simulink model "motorconfigmat"  (R2023b)
settings: Solver=VariableStepAuto  StartTime=0.0  StopTime=30  RelTol=1e-3
InitFcn:
  | Kpz = 0.3 ;
  | KIz = 0;
  | 
  | bh = 0.010290;  % batan hacim m^3
  | m = 10.5     ;  % aracın kütlesi kg
  | g = 9.81     ;  % yer çekimi ivmesi
  | p = 1000     ; % kg / m^3 yogunluk
  | W = m*g      ;  % aracın agırlıgı N
  | B = p*g*bh   ;  % Kaldırma kuvveti  N
  | 
  | xg = 0 ; % rgid body frame e göre ağırlık merkzi kordinatları
  | yg = 0 ;
  | zg = 0.02 ;
  | 
  | Ix = 0.1011 ; % kg *  m ^2
  | Iy = 0.1159 ;
  | Iz = 0.1615 ;
  | 
  | thrustCoefficient = 50/21.5 ;
  | 
  | % Add mass parametreleri
  | Xu_dot = -5.5;   % Surge direction
  | Yv_dot = -12.7;  % Sway direction
  | Zw_dot = -14.57; % Heave direction
  | 
  | Kp_dot = -0.12;  % Roll moment
  | Mq_dot = -0.12;  % Pitch moment
  | Nr_dot = -0.12;  % Yaw moment
  | 
  | % Linear Damping Values (Doğrusal Sönümleme Katsayıları)
  | Xu = -4.03;   % Ns/m
  | Yv = -6.22;   % Ns/m
  | Zw = -5.18;   % Ns/m
  | Kp = -0.07;   % Ns/rad
  | Mq = -0.07;   % Ns/rad
  | Nr = -0.07;   % Ns/rad
  | 
  | % Quadratic Damping Values (Doğrusal Olmayan Sönümleme Katsayıları)
  | Xuu = -18.18;  % Ns^2/m^2
  | Yvv = -21.66;  % Ns^2/m^2
  | Zww = -36.99;  % Ns^2/m^2
  | Kpp = -1.55;   % Ns^2/rad^2
  | Mqq = -1.55;   % Ns^2/rad^2
  | Nrr = -1.55;   % Ns^2/rad^2
undefined symbols (not defined in the file or in its folder): X, Y, Z
libraries: slpidlib x11, nesl_utility x7, sm_lib x6, fuzblock x1
(part 1 of 2)
settings Model: Creator=Yaser  LastModifiedBy=User

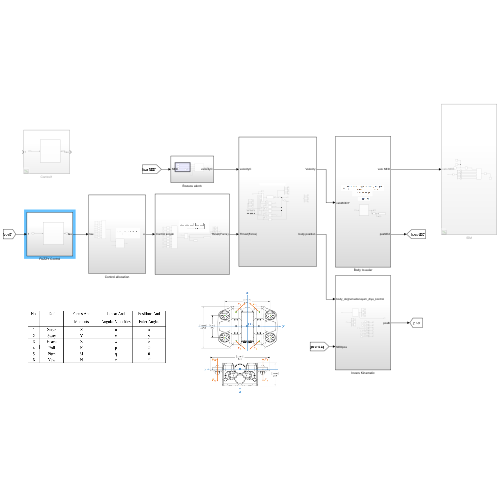
[thumbnail: Simulink's stored preview of the top-level diagram]
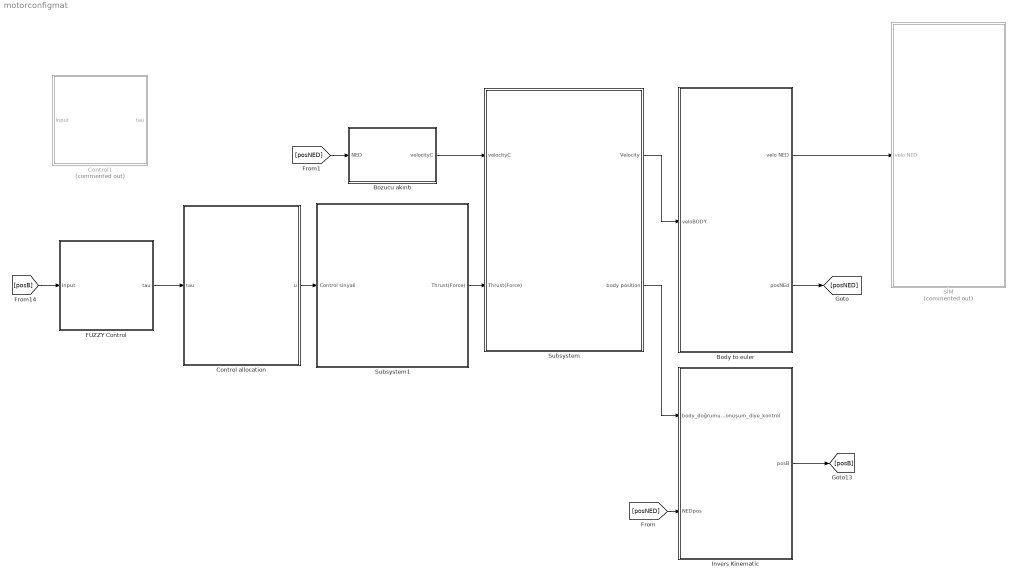
== system motorconfigmat ==
  Body to euler : Subsystem
  Bozucu akıntı : Subsystem
  Control allocation : Subsystem
  Control1 : Subsystem  Commented=on
  FUZZY Control : Subsystem
  Invers Kinematic : Subsystem
  Subsystem : Subsystem
  Subsystem1 : Subsystem
  SİM : Subsystem  Commented=on
  wires:
  [posNED] -> Invers Kinematic/2(NEDpos)
  Subsystem/2(body position) -> Invers Kinematic/1(body_doğrumudonuşum_diye_kontrol)
  Body to euler/2(posNEd) -> [posNED]
  [posB] -> FUZZY Control/1(Input)
  Subsystem/1(Velocity) -> Body to euler/1(veloBODY)
  Bozucu akıntı/1(velocityC) -> Subsystem/1(velocityC)
  Body to euler/1(velo NED) -> SİM/1(velo NED)
  Invers Kinematic/1(posB) -> [posB]
  Subsystem1/1(Thrust(Force)) -> Subsystem/2(Thrust(Force))
  FUZZY Control/1(tau) -> Control allocation/1(tau)
  Control allocation/1(u) -> Subsystem1/1(Control sinyali)
  [posNED] -> Bozucu akıntı/1(NED)

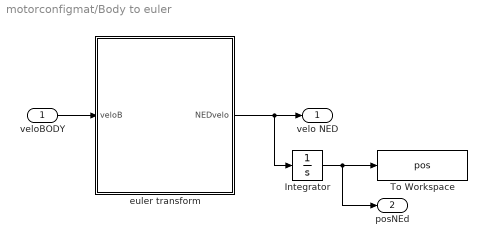
== system motorconfigmat/Body to euler ==
  veloBODY : Inport
  Integrator : Integrator
  To Workspace : ToWorkspace  VariableName=pos  SaveFormat=Timeseries  SampleTime=-1
  euler transform : MATLAB Function  TreatAsAtomicUnit=on
  velo NED : Outport
  posNEd : Outport  Port=2
  wires:
  veloBODY/1 -> euler transform/1(veloB)
  euler transform/1(NEDvelo) -> Integrator/1, velo NED/1
  Integrator/1 -> To Workspace/1, posNEd/1

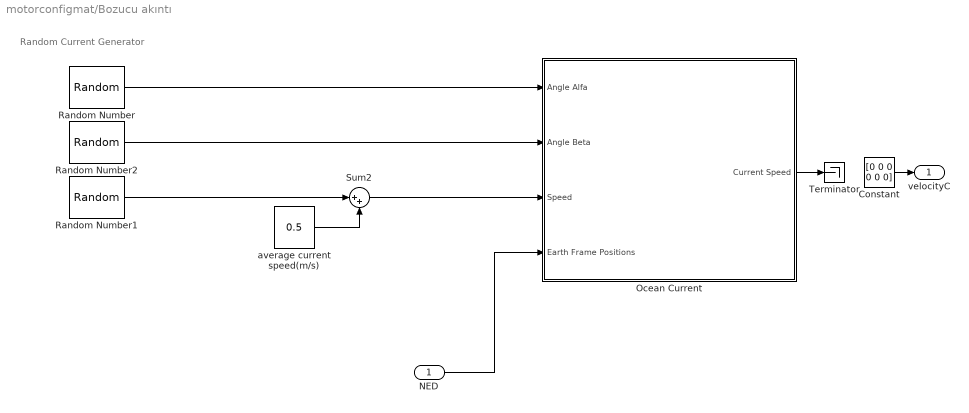
== system motorconfigmat/Bozucu akıntı ==
  note: Random Current Generator
  NED : Inport
  Constant : Constant  Value=[0 0 0 0 0 0]
  Ocean Current : Subsystem
  Random Number : RandomNumber  Mean=45  Variance=45  Seed=1  SampleTime=5
  Random Number1 : RandomNumber  Variance=0.02  Seed=0.025  SampleTime=5
  Random Number2 : RandomNumber  Mean=45  Variance=45  Seed=1  SampleTime=5
  Sum2 : Sum  Inputs=|++
  Terminator : Terminator
  average current speed(m/s) : Constant  Value=0.5
  velocityC : Outport
  wires:
  Random Number1/1 -> Sum2/1
  Random Number/1 -> Ocean Current/1(Angle Alfa)
  average current speed(m/s)/1 -> Sum2/2
  Sum2/1 -> Ocean Current/3(Speed)
  Random Number2/1 -> Ocean Current/2(Angle Beta)
  NED/1 -> Ocean Current/4(Earth Frame Positions)
  Ocean Current/1(Current Speed) -> Terminator/1
  Constant/1 -> velocityC/1

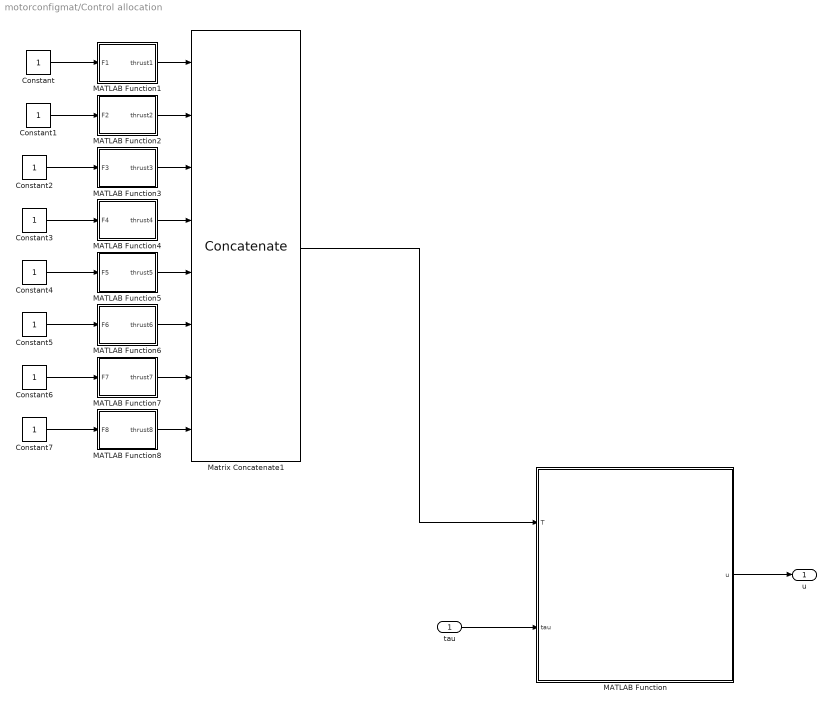
== system motorconfigmat/Control allocation ==
  tau : Inport
  Constant{,1..7} (8 alike) : Constant
  MATLAB Function : MATLAB Function  TreatAsAtomicUnit=on
  MATLAB Function1 : MATLAB Function  TreatAsAtomicUnit=on
  MATLAB Function2 : MATLAB Function  TreatAsAtomicUnit=on
  MATLAB Function3 : MATLAB Function  TreatAsAtomicUnit=on
  MATLAB Function4 : MATLAB Function  TreatAsAtomicUnit=on
  MATLAB Function5 : MATLAB Function  TreatAsAtomicUnit=on
  MATLAB Function6 : MATLAB Function  TreatAsAtomicUnit=on
  MATLAB Function7 : MATLAB Function  TreatAsAtomicUnit=on
  MATLAB Function8 : MATLAB Function  TreatAsAtomicUnit=on
  Matrix Concatenate1 : Concatenate  NumInputs=8  Mode=Multidimensional array  ConcatenateDimension=2
  u : Outport
  wires:
  MATLAB Function/1(u) -> u/1
  tau/1 -> MATLAB Function/2(tau)
  MATLAB Function4/1(thrust4) -> Matrix Concatenate1/4
  Constant/1 -> MATLAB Function1/1(F1)
  MATLAB Function2/1(thrust2) -> Matrix Concatenate1/2
  Constant6/1 -> MATLAB Function7/1(F7)
  MATLAB Function6/1(thrust6) -> Matrix Concatenate1/6
  MATLAB Function8/1(thrust8) -> Matrix Concatenate1/8
  Constant5/1 -> MATLAB Function6/1(F6)
  MATLAB Function7/1(thrust7) -> Matrix Concatenate1/7
  Constant4/1 -> MATLAB Function5/1(F5)
  Constant3/1 -> MATLAB Function4/1(F4)
  Constant7/1 -> MATLAB Function8/1(F8)
  MATLAB Function5/1(thrust5) -> Matrix Concatenate1/5
  Constant2/1 -> MATLAB Function3/1(F3)
  MATLAB Function3/1(thrust3) -> Matrix Concatenate1/3
  MATLAB Function1/1(thrust1) -> Matrix Concatenate1/1
  Constant1/1 -> MATLAB Function2/1(F2)
  Matrix Concatenate1/1 -> MATLAB Function/1(T)

== system motorconfigmat/Control1 ==
  Input : Inport
  divecont1 : Subsystem
  tau : Outport
  wires:
  divecont1/1(Out1) -> tau/1
  Input/1 -> divecont1/1(Input)

== system motorconfigmat/FUZZY Control ==
  Input : Inport
  divecont1 : Subsystem
  tau : Outport
  wires:
  Input/1 -> divecont1/1(Input)
  divecont1/1(Out1) -> tau/1

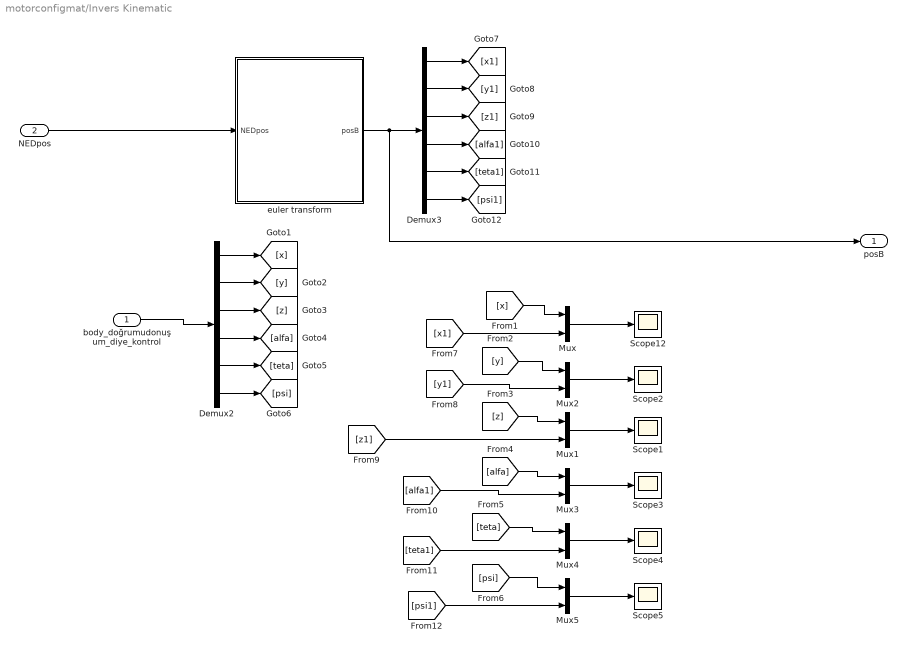
== system motorconfigmat/Invers Kinematic ==
  body_doğrumudonuşum_diye_kontrol : Inport
  NEDpos : Inport  Port=2
  Demux2 : Demux  Outputs=6
  Demux3 : Demux  Outputs=6
  Mux{,1..5} (6 alike) : Mux  Inputs=2
  Scope{1..5,12} (6 alike) : Scope
  euler transform : MATLAB Function  TreatAsAtomicUnit=on
  posB : Outport
  wires:
  [psi1] -> Mux5/2
  body_doğrumudonuşum_diye_kontrol/1 -> Demux2/1
  [x1] -> Mux/2
  Mux4/1 -> Scope4/1
  [z] -> Mux1/1
  euler transform/1(posB) -> posB/1, Demux3/1
  Demux3/1 -> [x1]
  Demux3/4 -> [alfa1]
  Demux3/5 -> [teta1]
  [z1] -> Mux1/2
  [y1] -> Mux2/2
  Mux3/1 -> Scope3/1
  [x] -> Mux/1
  Demux2/5 -> [teta]
  [psi] -> Mux5/1
  Demux3/6 -> [psi1]
  [alfa1] -> Mux3/2
  [teta1] -> Mux4/2
  [alfa] -> Mux3/1
  [teta] -> Mux4/1
  Mux2/1 -> Scope2/1
  Demux3/2 -> [y1]
  Demux2/1 -> [x]
  Mux1/1 -> Scope1/1
  [y] -> Mux2/1
  Demux3/3 -> [z1]
  Demux2/3 -> [z]
  Mux5/1 -> Scope5/1
  NEDpos/1 -> euler transform/1(NEDpos)
  Demux2/2 -> [y]
  Demux2/6 -> [psi]
  Mux/1 -> Scope12/1
  Demux2/4 -> [alfa]

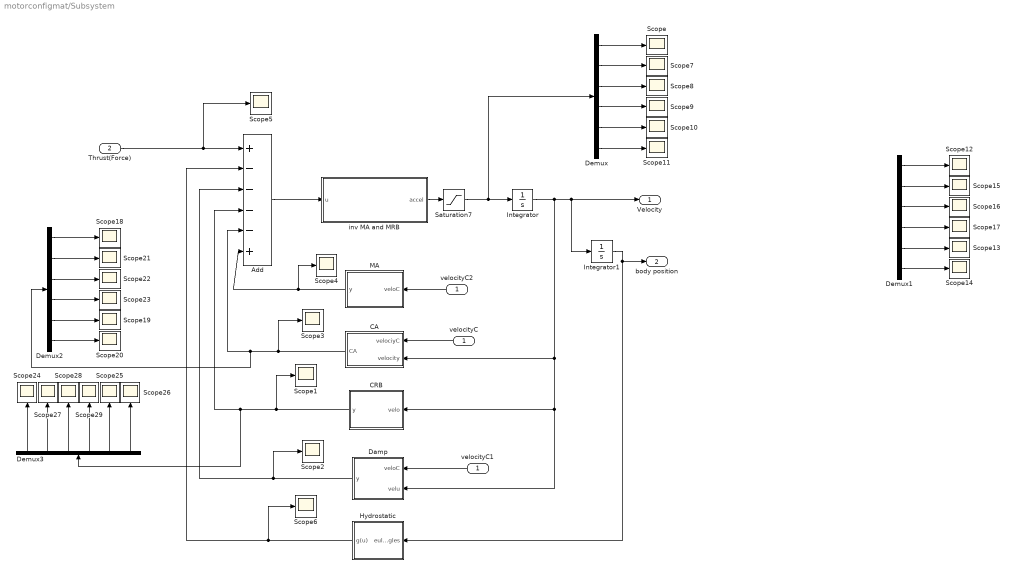
== system motorconfigmat/Subsystem ==
  velocityC : Inport
  Thrust(Force) : Inport  Port=2
  Add : Sum  Inputs=+----+
  CA : Subsystem
  CRB : Subsystem
  Damp : Subsystem
  Demux{,1..3} (4 alike) : Demux  Outputs=6
  Hydrostatic : Subsystem
  Integrator : Integrator
  Integrator1 : Integrator
  MA : Subsystem
  Saturation7 : Saturate  UpperLimit=1000  LowerLimit=-100
  Scope{,1..29} (30 alike) : Scope
  inv MA and MRB : Subsystem
  velocityC1 : InportShadow
  velocityC2 : InportShadow
  Velocity : Outport
  body position : Outport  Port=2
  wires:
  CA/1(CA) -> Scope3/1, Demux2/1, Add/5
  CRB/1(y) -> Scope1/1, Demux3/1, Add/4
  Integrator1/1 -> body position/1, Hydrostatic/1(euler angles)
  Add/1 -> inv MA and MRB/1(u)
  Integrator/1 -> Integrator1/1, Velocity/1, Damp/2(velu), CRB/1(velo), CA/2(velocity)
  Hydrostatic/1(g(u)) -> Scope6/1, Add/2
  Damp/1(y) -> Scope2/1, Add/3
  velocityC/1 -> CA/1(velociyC)
  velocityC1/1 -> Damp/1(veloC)
  velocityC2/1 -> MA/1(veloC)
  MA/1(y) -> Scope4/1, Add/6
  inv MA and MRB/1(accel) -> Saturation7/1
  Saturation7/1 -> Demux/1, Integrator/1
  Thrust(Force)/1 -> Scope5/1, Add/1
  Demux/1 -> Scope/1
  Demux/2 -> Scope7/1
  Demux/3 -> Scope8/1
  Demux/4 -> Scope9/1
  Demux/5 -> Scope10/1
  Demux/6 -> Scope11/1
  Demux1/1 -> Scope12/1
  Demux1/3 -> Scope16/1
  Demux1/6 -> Scope14/1
  Demux1/2 -> Scope15/1
  Demux1/4 -> Scope17/1
  Demux1/5 -> Scope13/1
  Demux2/1 -> Scope18/1
  Demux2/4 -> Scope23/1
  Demux2/2 -> Scope21/1
  Demux2/3 -> Scope22/1
  Demux2/5 -> Scope19/1
  Demux2/6 -> Scope20/1
  Demux3/5 -> Scope25/1
  Demux3/3 -> Scope28/1
  Demux3/2 -> Scope27/1
  Demux3/1 -> Scope24/1
  Demux3/4 -> Scope29/1
  Demux3/6 -> Scope26/1

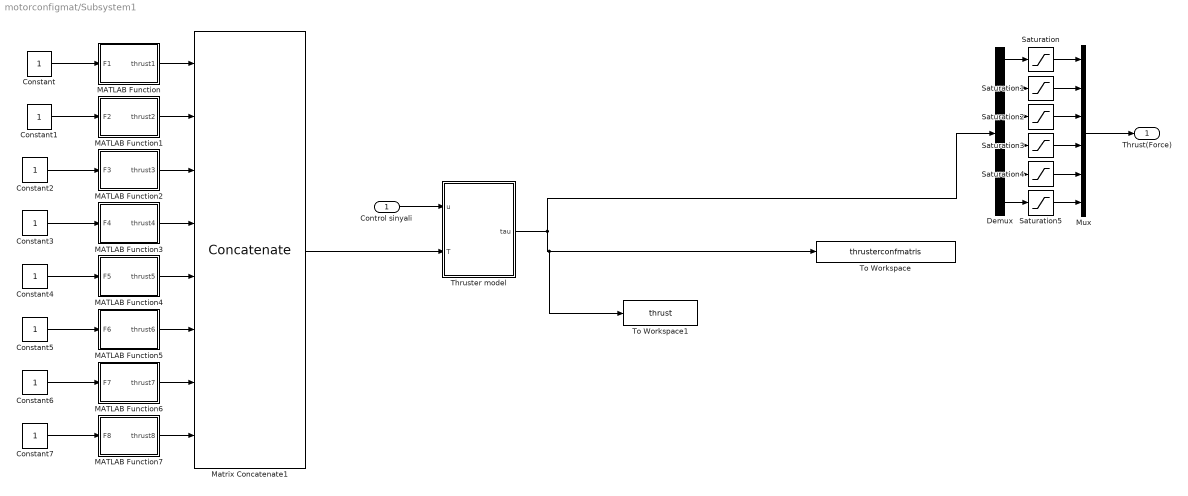
== system motorconfigmat/Subsystem1 ==
  Control sinyali : Inport
  Constant{,1..7} (8 alike) : Constant
  Demux : Demux  Outputs=6
  MATLAB Function : MATLAB Function  TreatAsAtomicUnit=on
  MATLAB Function1 : MATLAB Function  TreatAsAtomicUnit=on
  MATLAB Function2 : MATLAB Function  TreatAsAtomicUnit=on
  MATLAB Function3 : MATLAB Function  TreatAsAtomicUnit=on
  MATLAB Function4 : MATLAB Function  TreatAsAtomicUnit=on
  MATLAB Function5 : MATLAB Function  TreatAsAtomicUnit=on
  MATLAB Function6 : MATLAB Function  TreatAsAtomicUnit=on
  MATLAB Function7 : MATLAB Function  TreatAsAtomicUnit=on
  Matrix Concatenate1 : Concatenate  NumInputs=8  Mode=Multidimensional array  ConcatenateDimension=2
  Mux : Mux  Inputs=6
  Saturation : Saturate  UpperLimit=40*0.707*4  LowerLimit=-40*0.707*4
  Saturation1 : Saturate  UpperLimit=40*0.707*4  LowerLimit=-40*0.707*4
  Saturation2 : Saturate  UpperLimit=40*4  LowerLimit=-40*4
  Saturation3 : Saturate  UpperLimit=80*0.218*2  LowerLimit=-80*0.218*2
  Saturation4 : Saturate  UpperLimit=80*0.12*2  LowerLimit=-80*0.12*2
  Saturation5 : Saturate  UpperLimit=40*4*0.192  LowerLimit=-40*4*0.192
  Thruster model : MATLAB Function  TreatAsAtomicUnit=on
  To Workspace : ToWorkspace  VariableName=thrusterconfmatris  SaveFormat=Timeseries  SampleTime=-1
  To Workspace1 : ToWorkspace  VariableName=thrust  SaveFormat=Timeseries  SampleTime=-1
  Thrust(Force) : Outport
  wires:
  Thruster model/1(tau) -> To Workspace1/1, To Workspace/1, Demux/1
  Control sinyali/1 -> Thruster model/1(u)
  Matrix Concatenate1/1 -> Thruster model/2(T)
  Constant/1 -> MATLAB Function/1(F1)
  MATLAB Function/1(thrust1) -> Matrix Concatenate1/1
  Constant1/1 -> MATLAB Function1/1(F2)
  MATLAB Function1/1(thrust2) -> Matrix Concatenate1/2
  Constant2/1 -> MATLAB Function2/1(F3)
  Constant3/1 -> MATLAB Function3/1(F4)
  Constant4/1 -> MATLAB Function4/1(F5)
  Constant5/1 -> MATLAB Function5/1(F6)
  Constant6/1 -> MATLAB Function6/1(F7)
  Constant7/1 -> MATLAB Function7/1(F8)
  MATLAB Function7/1(thrust8) -> Matrix Concatenate1/8
  MATLAB Function6/1(thrust7) -> Matrix Concatenate1/7
  MATLAB Function5/1(thrust6) -> Matrix Concatenate1/6
  MATLAB Function4/1(thrust5) -> Matrix Concatenate1/5
  MATLAB Function3/1(thrust4) -> Matrix Concatenate1/4
  MATLAB Function2/1(thrust3) -> Matrix Concatenate1/3
  Saturation/1 -> Mux/1
  Saturation1/1 -> Mux/2
  Saturation2/1 -> Mux/3
  Saturation3/1 -> Mux/4
  Saturation4/1 -> Mux/5
  Saturation5/1 -> Mux/6
  Mux/1 -> Thrust(Force)/1
  Demux/1 -> Saturation/1
  Demux/2 -> Saturation1/1
  Demux/3 -> Saturation2/1
  Demux/4 -> Saturation3/1
  Demux/5 -> Saturation4/1
  Demux/6 -> Saturation5/1

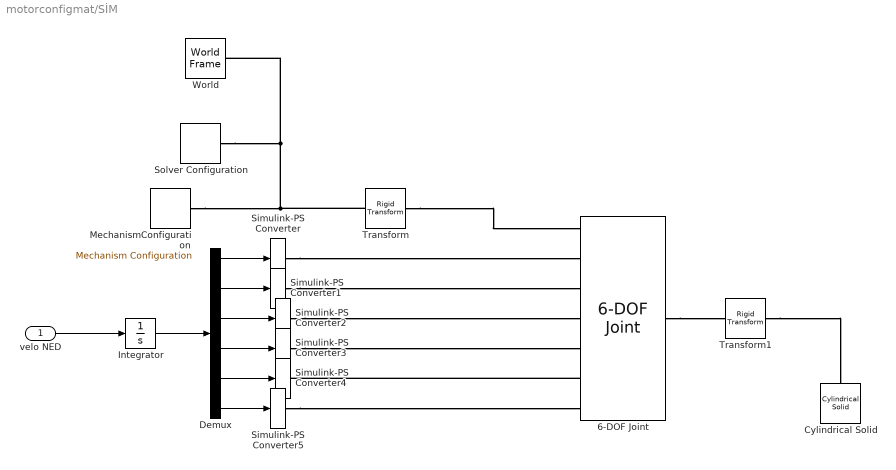
== system motorconfigmat/SİM ==
  velo NED : Inport
  6-DOF Joint : sm_lib/Joints/6-DOF Joint  JointMode=Normal  SenseConstraintForce=off  SenseConstraintForceX=off  SenseConstraintForceY=off  SenseConstraintForceZ=off  SenseConstraintTorque=off  SenseConstraintTorqueX=off  SenseConstraintTorqueY=off  SenseConstraintTorqueZ=off  SenseTotalForce=off  SenseTotalForceX=off  SenseTotalForceY=off  SenseTotalForceZ=off  SenseTotalTorque=off  SenseTotalTorqueX=off  SenseTotalTorqueY=off  SenseTotalTorqueZ=off  CompositeWrenchDir=FollowerOnBase  CompositeWrenchFrame=BaseFrame  PxEquilibriumPosition=0  PxEquilibriumPositionUnits=m  PxSpringStiffness=0  PxSpringStiffnessUnits=N/m  PxDampingCoefficient=0  PxDampingCoefficientUnits=N/(m/s)  PxTorqueActuationMode=ComputedTorque  PxMotionActuationMode=InputMotion  PxSensePosition=off  PxSenseVelocity=off  PxSenseAcceleration=off  PxSenseTorqueForce=off  PxSenseLowerLimitTorqueForce=off  PxSenseUpperLimitTorqueForce=off  PxLowerLimitSpecify=off  PxLowerLimitBound=-1  PxLowerLimitBoundUnits=m  PxLowerLimitStiffness=1e6  PxLowerLimitStiffnessUnits=N/m  PxLowerLimitDamping=1e3  PxLowerLimitDampingUnits=N/(m/s)  PxLowerLimitTransitionRegionWidth=1e-4  PxLowerLimitTransitionRegionWidthUnits=m  PxUpperLimitSpecify=off  PxUpperLimitBound=1  PxUpperLimitBoundUnits=m  PxUpperLimitStiffness=1e6  PxUpperLimitStiffnessUnits=N/m  PxUpperLimitDamping=1e3  PxUpperLimitDampingUnits=N/(m/s)  PxUpperLimitTransitionRegionWidth=1e-4  PxUpperLimitTransitionRegionWidthUnits=m  PxPositionTargetSpecify=off  PxPositionTargetPriority=High  PxPositionTargetValue=0  PxPositionTargetValueUnits=m  PxVelocityTargetSpecify=off  PxVelocityTargetPriority=High  PxVelocityTargetValue=0  PxVelocityTargetValueUnits=m/s  PyEquilibriumPosition=0  PyEquilibriumPositionUnits=m  PySpringStiffness=0  PySpringStiffnessUnits=N/m  PyDampingCoefficient=0  PyDampingCoefficientUnits=N/(m/s)  PyTorqueActuationMode=ComputedTorque  PyMotionActuationMode=InputMotion  PySensePosition=off  PySenseVelocity=off  PySenseAcceleration=off  PySenseTorqueForce=off  PySenseLowerLimitTorqueForce=off  PySenseUpperLimitTorqueForce=off  PyLowerLimitSpecify=off  PyLowerLimitBound=-1  PyLowerLimitBoundUnits=m  PyLowerLimitStiffness=1e6  PyLowerLimitStiffnessUnits=N/m  PyLowerLimitDamping=1e3  PyLowerLimitDampingUnits=N/(m/s)  PyLowerLimitTransitionRegionWidth=1e-4  PyLowerLimitTransitionRegionWidthUnits=m  PyUpperLimitSpecify=off  PyUpperLimitBound=1  PyUpperLimitBoundUnits=m  PyUpperLimitStiffness=1e6  PyUpperLimitStiffnessUnits=N/m  PyUpperLimitDamping=1e3  PyUpperLimitDampingUnits=N/(m/s)  PyUpperLimitTransitionRegionWidth=1e-4  PyUpperLimitTransitionRegionWidthUnits=m  PyPositionTargetSpecify=off  PyPositionTargetPriority=High  PyPositionTargetValue=0  PyPositionTargetValueUnits=m  PyVelocityTargetSpecify=off  PyVelocityTargetPriority=High  PyVelocityTargetValue=0  PyVelocityTargetValueUnits=m/s  PzEquilibriumPosition=0  PzEquilibriumPositionUnits=m  PzSpringStiffness=0  PzSpringStiffnessUnits=N/m  PzDampingCoefficient=0  PzDampingCoefficientUnits=N/(m/s)  PzTorqueActuationMode=ComputedTorque  PzMotionActuationMode=InputMotion  PzSensePosition=off  PzSenseVelocity=off  PzSenseAcceleration=off  PzSenseTorqueForce=off  PzSenseLowerLimitTorqueForce=off  PzSenseUpperLimitTorqueForce=off  PzLowerLimitSpecify=off  PzLowerLimitBound=-1  PzLowerLimitBoundUnits=m  PzLowerLimitStiffness=1e6  PzLowerLimitStiffnessUnits=N/m  PzLowerLimitDamping=1e3  PzLowerLimitDampingUnits=N/(m/s)  PzLowerLimitTransitionRegionWidth=1e-4  PzLowerLimitTransitionRegionWidthUnits=m  PzUpperLimitSpecify=off  PzUpperLimitBound=1  PzUpperLimitBoundUnits=m  PzUpperLimitStiffness=1e6  PzUpperLimitStiffnessUnits=N/m  PzUpperLimitDamping=1e3  PzUpperLimitDampingUnits=N/(m/s)  PzUpperLimitTransitionRegionWidth=1e-4  PzUpperLimitTransitionRegionWidthUnits=m  PzPositionTargetSpecify=off  PzPositionTargetPriority=High  PzPositionTargetValue=0  PzPositionTargetValueUnits=m  PzVelocityTargetSpecify=off  PzVelocityTargetPriority=High  PzVelocityTargetValue=0  PzVelocityTargetValueUnits=m/s  SphEqPosRotationMethod=None  SphEqPosRotationAngleUnits=deg  SphEqPosRotationStandardAxis=+Z  SphEqPosRotationAngle=0  SphEqPosRotationArbitraryAxis=[0 0 1]  SphEqPosFollAlignAxisA=+X  SphEqPosBaseAlignAxisA=+Y  SphEqPosFollAlignAxisB=+Y  SphEqPosBaseAlignAxisB=+Z  SphEqPosRotationSequenceAxes=FollowerAxes  SphEqPosRotationSequence=XYX  SphEqPosRotationSequenceAngles=[0 0 0]  SphEqPosRotationSequenceAnglesUnits=deg  SphEqPosRotationMatrix=[1 0 0;0 1 0;0 0 1]  SphEqPosQuaternion=[1 0 0 0]  SphSpringStiffness=0  SphSpringStiffnessUnits=N*m/deg  SphDampingCoefficient=0  SphDampingCoefficientUnits=N*m/(deg/s)  SphActuateTorqueX=on  SphActuateTorqueY=on  SphActuateTorqueZ=on  SphActuateTorque=off  SphTorqueActuationMode=InputTorque  SphMotionActuationMode=ComputedMotion  SphActuationFrame=BaseFrame  SphSensePosition=off  SphSenseVelocityX=off  SphSenseVelocityY=off  SphSenseVelocityZ=off  SphSenseVelocity=off  SphSenseAccelerationX=off  SphSenseAccelerationY=off  SphSenseAccelerationZ=off  SphSenseAcceleration=off  SphSenseTorqueX=off  SphSenseTorqueY=off  SphSenseTorqueZ=off  SphSenseTorqueForce=off  SphSenseLowerLimitTorqueMag=off  SphSenseUpperLimitTorqueMag=off  SphSensingFrame=BaseFrame  SphLowerLimitSpecify=off  SphLowerLimitBound=15  SphLowerLimitBoundUnits=deg  SphLowerLimitStiffness=1e4  SphLowerLimitStiffnessUnits=N*m/deg  SphLowerLimitDamping=10  SphLowerLimitDampingUnits=N*m/(deg/s)  SphLowerLimitTransitionRegionWidth=0.1  SphLowerLimitTransitionRegionWidthUnits=deg  SphUpperLimitSpecify=off  SphUpperLimitBound=45  SphUpperLimitBoundUnits=deg  SphUpperLimitStiffness=1e4  SphUpperLimitStiffnessUnits=N*m/deg  SphUpperLimitDamping=10  SphUpperLimitDampingUnits=N*m/(deg/s)  SphUpperLimitTransitionRegionWidth=0.1  SphUpperLimitTransitionRegionWidthUnits=deg  SphPositionTargetRotationMethod=None  SphPositionTargetRotationAngleUnits=deg  SphPositionTargetRotationStandardAxis=+Z  SphPositionTargetRotationAngle=0  SphPositionTargetRotationArbitraryAxis=[0 0 1]  SphPositionTargetFollAlignAxisA=+X  SphPositionTargetBaseAlignAxisA=+Y  SphPositionTargetFollAlignAxisB=+Y  SphPositionTargetBaseAlignAxisB=+Z  SphPositionTargetRotationSequenceAxes=FollowerAxes  SphPositionTargetRotationSequence=XYX  SphPositionTargetRotationSequenceAngles=[0 0 0]  SphPositionTargetRotationSequenceAnglesUnits=deg  SphPositionTargetRotationMatrix=[1 0 0;0 1 0;0 0 1]  SphPositionTargetQuaternion=[1 0 0 0]  SphPositionTargetSpecify=off  SphPositionTargetPriority=High  SphVelocityTargetValue=[0 0 0]  SphVelocityTargetValueUnits=deg/s  SphVelocityTargetSpecify=off  SphVelocityTargetPriority=High  SphVelocityTargetInFollowerFrame=on
  Cylindrical Solid : sm_lib/Body Elements/Cylindrical Solid  GraphicAmbientColor=[0.15 0.15 0.15 1.0]  BasedOnType=Density  CenterOfMass=[0 0 0]  CenterOfMassUnits=m  GraphicDiffuseColor=[0.5 0.5 0.5]  CylinderLength=1  CylinderLengthUnits=m  CylinderRadius=1  CylinderRadiusUnits=m  Density=1000  DensityUnits=kg/m^3  DoExposeReferenceFrame=on  GraphicEmissiveColor=[0.0 0.0 0.0 1.0]  ExportEntireGeometry=off  SerializedFrames=<Frames/>  MarkerShape=Sphere  MarkerSize=10  GraphicType=FromGeometry  InertiaType=CalculateFromGeometry  Mass=1  MassUnits=kg  MomentsOfInertia=[1 1 1]  MomentsOfInertiaUnits=kg*m^2  GraphicOpacity=1.0  ProductsOfInertia=[0 0 0]  ProductsOfInertiaUnits=kg*m^2  GraphicShininess=75  GraphicSpecularColor=[0.5 0.5 0.5 1.0]  GraphicVisPropType=SimpleVisualProperties
  Demux : Demux  Outputs=6
  Integrator : Integrator
  MechanismConfiguration : sm_lib/Utilities/Mechanism Configuration  UniformGravity=Constant  GravityVector=[0 -9.8 0]  GravityVectorUnits=m/s^2  LinearizationDelta=0.001  JointModeTransitionNonlinearIterations=2
  Simulink-PS Converter{,1..5} (6 alike) : nesl_utility/Simulink-PS Converter  PhysicalDomain=network_engine_domain  SubClassName=ps_input  LeftPortType=input  RightPortType=output  PseudoPeriodic=off  Frequencies=[]  NoiseDistribution=none  NoiseParameters=[]  Unit=1  AffineConversion=off  FilteringAndDerivatives=filter  SimscapeFilterOrder=2  InputFilterTimeConstant=0.001  UdotUserProvided=0
  Solver Configuration : nesl_utility/Solver Configuration  PhysicalDomain=network_engine_domain  SubClassName=solver  LeftPortType=input  RightPortType=generic  Tones=[]  Harmonics=[]  SimulateNoise=off  Profile=off  UseLocalSampling=off  EnableSwitchedLinearOptims=on  FrequencyDomain=off  UseCCode=off  RelTol=0.001  AbsTol=0.001  MinStep=1e-09  ToWorkspace=off  RevertToSquareIcSolve=off  NumHomotopyIterations=100  PhasorMode=off  PhasorModeNumHarmonics=1  ConsistencySolver=NEWTON_XTOL_AFTER_FTOL  IndexReductionMethod=DerivativeReplacement  DoDC=off  ResidualTolerance=1e-09  ConsistencyTolSource=GLOBAL  ConsistencyAbsTol=0.001  ConsistencyRelTol=0.001  ConsistencyTolFactor=0.001  UseLocalSolver=off  LocalSolverChoice=NE_BACKWARD_EULER_ADVANCER  ResolveIndetEquations=on  FunctionEvalNumThread=1  LocalSolverSampleTime=0.001  DoFixedCost=off  MaxNonlinIter=3  MaxModeIter=2  ComputeImpulses=off  ImpulseIterations=2  LinearAlgebra=auto  LinearAlgebraNumThread=0  EquationFormulation=NE_TIME_EF  DelaysMemoryBudget=1024  AutomaticFiltering=on  FilteringTimeConstant=0.001  PartitionStorageMethod=AS_NEEDED  PartitionMemoryBudget=1024  PartitionMethod=ROBUST  MultibodyUseLocalSolver=off  MultibodyLocalSolverChoice=ODE1  MultibodyLocalSolverSampleTime=0.001
  Transform : sm_lib/Frames and Transforms/Rigid Transform  TranslationMethod=None  TranslationStandardOffset=0  TranslationStandardOffsetUnits=m  TranslationStandardAxis=+Z  TranslationCartesianOffset=0  TranslationCartesianOffsetUnits=mm  TranslationROffset=0  TranslationROffsetUnits=m  TranslationZOffset=0  TranslationZOffsetUnits=m  TranslationThetaOffset=0  TranslationThetaOffsetUnits=deg  RotationMethod=ArbitraryAxis  RotationAngleUnits=rad  RotationStandardAxis=+Z  RotationAngle=0  RotationArbitraryAxis=[0,0,0]  FollAlignAxisA=+X  BaseAlignAxisA=+Y  FollAlignAxisB=+Y  BaseAlignAxisB=+Z  RotationSequenceAxes=FollowerAxes  RotationSequence=XYX  RotationSequenceAngles=[0 0 0]  RotationSequenceAnglesUnits=deg  RotationMatrix=[1 0 0;0 1 0;0 0 1]  Quaternion=[1 0 0 0]
  Transform1 : sm_lib/Frames and Transforms/Rigid Transform  TranslationMethod=None  TranslationStandardOffset=0  TranslationStandardOffsetUnits=m  TranslationStandardAxis=+Z  TranslationCartesianOffset=0  TranslationCartesianOffsetUnits=mm  TranslationROffset=0  TranslationROffsetUnits=m  TranslationZOffset=0  TranslationZOffsetUnits=m  TranslationThetaOffset=0  TranslationThetaOffsetUnits=deg  RotationMethod=ArbitraryAxis  RotationAngleUnits=rad  RotationStandardAxis=+Z  RotationAngle=0  RotationArbitraryAxis=[0,0,0]  FollAlignAxisA=+X  BaseAlignAxisA=+Y  FollAlignAxisB=+Y  BaseAlignAxisB=+Z  RotationSequenceAxes=FollowerAxes  RotationSequence=XYX  RotationSequenceAngles=[0 0 0]  RotationSequenceAnglesUnits=deg  RotationMatrix=[1 0 0;0 1 0;0 0 1]  Quaternion=[1 0 0 0]
  World : sm_lib/Frames and Transforms/World Frame
  wires:
  velo NED/1 -> Integrator/1
  Integrator/1 -> Demux/1
  Demux/1 -> Simulink-PS Converter/1
  Demux/2 -> Simulink-PS Converter1/1
  Demux/3 -> Simulink-PS Converter2/1
  Demux/4 -> Simulink-PS Converter3/1
  Demux/5 -> Simulink-PS Converter4/1
  Demux/6 -> Simulink-PS Converter5/1
  connections:
  Solver Configuration/RConn1 -- Transform/LConn1 -- MechanismConfiguration/RConn1 -- World/RConn1
  Simulink-PS Converter/RConn1 -- 6-DOF Joint/LConn2
  Simulink-PS Converter1/RConn1 -- 6-DOF Joint/LConn3
  Simulink-PS Converter3/RConn1 -- 6-DOF Joint/LConn5
  Simulink-PS Converter2/RConn1 -- 6-DOF Joint/LConn4
  Simulink-PS Converter5/RConn1 -- 6-DOF Joint/LConn7
  6-DOF Joint/LConn6 -- Simulink-PS Converter4/RConn1
  Transform/RConn1 -- 6-DOF Joint/LConn1
  Transform1/RConn1 -- Cylindrical Solid/RConn1
  6-DOF Joint/RConn1 -- Transform1/LConn1

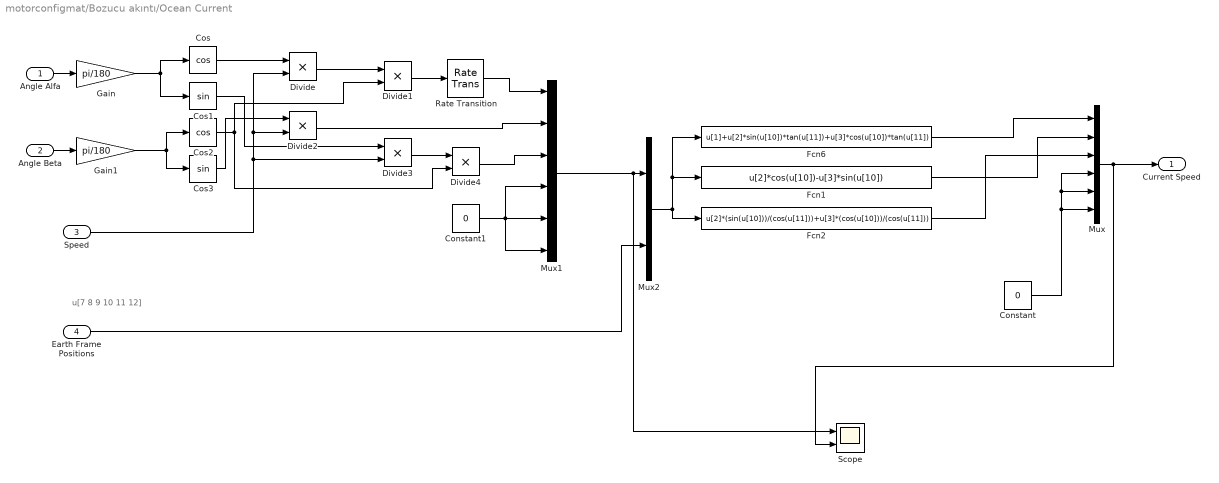
== system motorconfigmat/Bozucu akıntı/Ocean Current ==
  note: u[7 8 9 10 11 12]
  Angle Alfa : Inport
  Angle Beta : Inport  Port=2
  Speed : Inport  Port=3
  Earth Frame Positions : Inport  Port=4
  Constant : Constant  Value=0
  Constant1 : Constant  Value=0
  Cos : Trigonometry  Operator=cos
  Cos1 : Trigonometry
  Cos2 : Trigonometry  Operator=cos
  Cos3 : Trigonometry
  Divide{,1..4} (5 alike) : Product  Inputs=**
  Fcn1 : Fcn  Expr=u[2]*cos(u[10])-u[3]*sin(u[10])
  Fcn2 : Fcn  Expr=u[2]*(sin(u[10]))/(cos(u[11]))+u[3]*(cos(u[10]))/(cos(u[11]))
  Fcn6 : Fcn  Expr=u[1]+u[2]*sin(u[10])*tan(u[11])+u[3]*cos(u[10])*tan(u[11])
  Gain : Gain  Gain=pi/180
  Gain1 : Gain  Gain=pi/180
  Mux : Mux  Inputs=6
  Mux1 : Mux  Inputs=6
  Mux2 : Mux  Inputs=2
  Rate Transition : RateTransition
  Scope : Scope  NumInputPorts=2
  Current Speed : Outport
  wires:
  Angle Alfa/1 -> Gain/1
  Gain/1 -> Cos/1, Cos1/1
  Mux/1 -> Current Speed/1, Scope/2
  Constant/1 -> Mux/6, Mux/5, Mux/4
  Angle Beta/1 -> Gain1/1
  Gain1/1 -> Cos3/1, Cos2/1
  Cos/1 -> Divide/1
  Speed/1 -> Divide3/2, Divide2/2, Divide/2
  Cos2/1 -> Divide4/2, Divide1/2
  Divide/1 -> Divide1/1
  Divide1/1 -> Rate Transition/1
  Cos3/1 -> Divide2/1
  Divide2/1 -> Mux1/2
  Cos1/1 -> Divide3/1
  Divide3/1 -> Divide4/1
  Divide4/1 -> Mux1/3
  Constant1/1 -> Mux1/4, Mux1/6, Mux1/5
  Mux1/1 -> Scope/1, Mux2/1
  Earth Frame Positions/1 -> Mux2/2
  Mux2/1 -> Fcn1/1, Fcn6/1, Fcn2/1
  Fcn6/1 -> Mux/1
  Fcn1/1 -> Mux/2
  Fcn2/1 -> Mux/3
  Rate Transition/1 -> Mux1/1

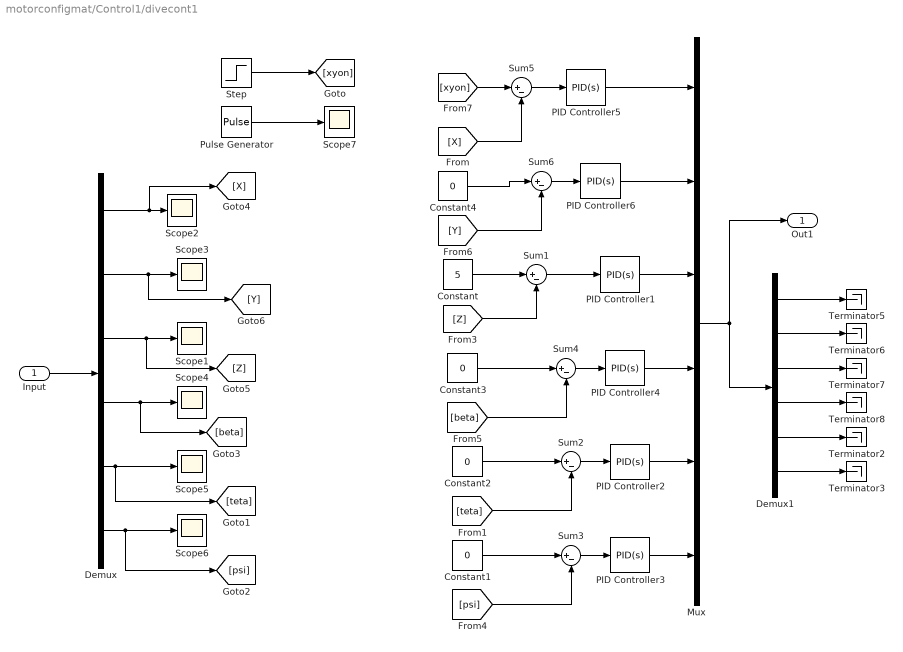
== system motorconfigmat/Control1/divecont1 ==
  Input : Inport
  Constant : Constant  Value=5
  Constant{1..4} (4 alike) : Constant  Value=0
  Demux : Demux  Outputs=6
  Demux1 : Demux  Outputs=6
  Mux : Mux  Inputs=6
  PID Controller1 : slpidlib/PID Controller  Controller=PID  Form=Parallel  TimeDomain=Continuous-time  UseExternalTs=off  SampleTime=-1  IntegratorMethod=Forward Euler  FilterMethod=Forward Euler  ControllerParametersSource=internal  P=2  I=0  UseKiTs=off  D=0  N=100  UseFilter=on  TunerSelectOption=Transfer Function Based (PID Tuner App)  InitialConditionSource=internal  InitialConditionForIntegrator=0  InitialConditionForFilter=0  DifferentiatorICPrevScaledInput=0  ExternalReset=none  TrackingMode=off  Kt=1  LimitOutput=off  SatLimitsSource=internal  UpperSaturationLimit=inf  LowerSaturationLimit=-inf  LinearizeAsGain=on  AntiWindupMode=none  Kb=1  LimitIntegrator=off  UpperIntegratorSaturationLimit=inf  LowerIntegratorSaturationLimit=-inf  POutMin=[]  POutMax=[]  IOutMin=[]  IOutMax=[]  DOutMin=[]  DOutMax=[]  NOutMin=[]  NOutMax=[]  SumOutMin=[]  SumOutMax=[]  SaturationOutMin=[]  SaturationOutMax=[]  PParamMin=[]  PParamMax=[]  IParamMin=[]  IParamMax=[]  DParamMin=[]  DParamMax=[]  NParamMin=[]  NParamMax=[]  KbParamMin=[]  KbParamMax=[]  KtParamMin=[]  KtParamMax=[]  KbOutMin=[]  KbOutMax=[]  KtOutMin=[]  KtOutMax=[]  IntegratorOutMin=[]  IntegratorOutMax=[]  FilterOutMin=[]  FilterOutMax=[]  SumI1OutMin=[]  SumI1OutMax=[]  SumI2OutMin=[]  SumI2OutMax=[]  SumI3OutMin=[]  SumI3OutMax=[]  SumI4OutMin=[]  SumI4OutMax=[]  SumDOutMin=[]  SumDOutMax=[]  DifferentiatorOutMin=[]  DifferentiatorOutMax=[]  FilterDiffOutCoefMin=[]  FilterDiffOutCoefMax=[]  ReciprocalOutMin=[]  ReciprocalOutMax=[]  SumDenOutMin=[]  SumDenOutMax=[]  SumNumOutMin=[]  SumNumOutMax=[]  DivideOutMin=[]  DivideOutMax=[]  UdiffTsProdOutMin=[]  UdiffTsProdOutMax=[]  NTsProdOutMin=[]  NTsProdOutMax=[]  UintegralTsProdOutMin=[]  UintegralTsProdOutMax=[]  UngainTsProdOutMin=[]  UngainTsProdOutMax=[]  ClampingZeroOutDataTypeStr=Inherit: Inherit via back propagation  ClampingZeroOutMin=[]  ClampingZeroOutMax=[]  FilterDenConstantOutDataTypeStr=Inherit: Inherit via back propagation  FilterDenConstantOutMin=[]  FilterDenConstantOutMax=[]  PCopyOutDataTypeStr=Inherit: Inherit via back propagation  PCopyOutMin=[]  PCopyOutMax=[]  NCopyOutDataTypeStr=Inherit: Inherit via back propagation  NCopyOutMin=[]  NCopyOutMax=[]  IntegratorContinuousStateAttributes=''  IntegratorStateMustResolveToSignalObject=off  IntegratorRTWStateStorageClass=Auto  FilterContinuousStateAttributes=''  FilterStateMustResolveToSignalObject=off  FilterRTWStateStorageClass=Auto  ParallelPVariant=InternalParameters  IdealPVariant=Disabled  IVariant=InternalParameters  DVariant=InternalParameters  IntegratorVariant=Continuous  SatVariant=Disabled  AWVariant=Passthrough  PCopyVariant=Disabled  TRVariant=Disabled  FdbkBlocksVariant=Forward  IdealPFdbkVariant=Disabled  SatFdbkVariant=Disabled  DerivativeFilterVariant=ContFilter  NVariant=InternalParameters  NCopyVariant=Disabled  FilterICVariant=InternalICsFilter  IntegratorICVariant=InternalICs  ExternalResetVariant=Disabled  TRSumVariant=Passthrough  SumFdbkVariant=Disabled  SumVariant=Sum_PID  TsampFilterVariant=InternalTs  TsampNgainVariant=Passthrough  TsampIntegralVariant=Disabled_SignalSpec  ExternalSaturationOutDataTypeStr=Inherit: Same as second input
  PID Controller{2..4,6} (4 alike) : slpidlib/PID Controller  Controller=PID  Form=Parallel  TimeDomain=Continuous-time  UseExternalTs=off  SampleTime=-1  IntegratorMethod=Forward Euler  FilterMethod=Forward Euler  ControllerParametersSource=internal  P=0.2  I=0  UseKiTs=off  D=0  N=100  UseFilter=on  TunerSelectOption=Transfer Function Based (PID Tuner App)  InitialConditionSource=internal  InitialConditionForIntegrator=0  InitialConditionForFilter=0  DifferentiatorICPrevScaledInput=0  ExternalReset=none  TrackingMode=off  Kt=1  LimitOutput=off  SatLimitsSource=internal  UpperSaturationLimit=inf  LowerSaturationLimit=-inf  LinearizeAsGain=on  AntiWindupMode=none  Kb=1  LimitIntegrator=off  UpperIntegratorSaturationLimit=inf  LowerIntegratorSaturationLimit=-inf  POutMin=[]  POutMax=[]  IOutMin=[]  IOutMax=[]  DOutMin=[]  DOutMax=[]  NOutMin=[]  NOutMax=[]  SumOutMin=[]  SumOutMax=[]  SaturationOutMin=[]  SaturationOutMax=[]  PParamMin=[]  PParamMax=[]  IParamMin=[]  IParamMax=[]  DParamMin=[]  DParamMax=[]  NParamMin=[]  NParamMax=[]  KbParamMin=[]  KbParamMax=[]  KtParamMin=[]  KtParamMax=[]  KbOutMin=[]  KbOutMax=[]  KtOutMin=[]  KtOutMax=[]  IntegratorOutMin=[]  IntegratorOutMax=[]  FilterOutMin=[]  FilterOutMax=[]  SumI1OutMin=[]  SumI1OutMax=[]  SumI2OutMin=[]  SumI2OutMax=[]  SumI3OutMin=[]  SumI3OutMax=[]  SumI4OutMin=[]  SumI4OutMax=[]  SumDOutMin=[]  SumDOutMax=[]  DifferentiatorOutMin=[]  DifferentiatorOutMax=[]  FilterDiffOutCoefMin=[]  FilterDiffOutCoefMax=[]  ReciprocalOutMin=[]  ReciprocalOutMax=[]  SumDenOutMin=[]  SumDenOutMax=[]  SumNumOutMin=[]  SumNumOutMax=[]  DivideOutMin=[]  DivideOutMax=[]  UdiffTsProdOutMin=[]  UdiffTsProdOutMax=[]  NTsProdOutMin=[]  NTsProdOutMax=[]  UintegralTsProdOutMin=[]  UintegralTsProdOutMax=[]  UngainTsProdOutMin=[]  UngainTsProdOutMax=[]  ClampingZeroOutDataTypeStr=Inherit: Inherit via back propagation  ClampingZeroOutMin=[]  ClampingZeroOutMax=[]  FilterDenConstantOutDataTypeStr=Inherit: Inherit via back propagation  FilterDenConstantOutMin=[]  FilterDenConstantOutMax=[]  PCopyOutDataTypeStr=Inherit: Inherit via back propagation  PCopyOutMin=[]  PCopyOutMax=[]  NCopyOutDataTypeStr=Inherit: Inherit via back propagation  NCopyOutMin=[]  NCopyOutMax=[]  IntegratorContinuousStateAttributes=''  IntegratorStateMustResolveToSignalObject=off  IntegratorRTWStateStorageClass=Auto  FilterContinuousStateAttributes=''  FilterStateMustResolveToSignalObject=off  FilterRTWStateStorageClass=Auto  ParallelPVariant=InternalParameters  IdealPVariant=Disabled  IVariant=InternalParameters  DVariant=InternalParameters  IntegratorVariant=Continuous  SatVariant=Disabled  AWVariant=Passthrough  PCopyVariant=Disabled  TRVariant=Disabled  FdbkBlocksVariant=Forward  IdealPFdbkVariant=Disabled  SatFdbkVariant=Disabled  DerivativeFilterVariant=ContFilter  NVariant=InternalParameters  NCopyVariant=Disabled  FilterICVariant=InternalICsFilter  IntegratorICVariant=InternalICs  ExternalResetVariant=Disabled  TRSumVariant=Passthrough  SumFdbkVariant=Disabled  SumVariant=Sum_PID  TsampFilterVariant=InternalTs  TsampNgainVariant=Passthrough  TsampIntegralVariant=Disabled_SignalSpec  ExternalSaturationOutDataTypeStr=Inherit: Same as second input
  PID Controller5 : slpidlib/PID Controller  Controller=PID  Form=Parallel  TimeDomain=Continuous-time  UseExternalTs=off  SampleTime=-1  IntegratorMethod=Forward Euler  FilterMethod=Forward Euler  ControllerParametersSource=internal  P=0.9  I=0  UseKiTs=off  D=0  N=100  UseFilter=on  TunerSelectOption=Transfer Function Based (PID Tuner App)  InitialConditionSource=internal  InitialConditionForIntegrator=0  InitialConditionForFilter=0  DifferentiatorICPrevScaledInput=0  ExternalReset=none  TrackingMode=off  Kt=1  LimitOutput=off  SatLimitsSource=internal  UpperSaturationLimit=inf  LowerSaturationLimit=-inf  LinearizeAsGain=on  AntiWindupMode=none  Kb=1  LimitIntegrator=off  UpperIntegratorSaturationLimit=inf  LowerIntegratorSaturationLimit=-inf  POutMin=[]  POutMax=[]  IOutMin=[]  IOutMax=[]  DOutMin=[]  DOutMax=[]  NOutMin=[]  NOutMax=[]  SumOutMin=[]  SumOutMax=[]  SaturationOutMin=[]  SaturationOutMax=[]  PParamMin=[]  PParamMax=[]  IParamMin=[]  IParamMax=[]  DParamMin=[]  DParamMax=[]  NParamMin=[]  NParamMax=[]  KbParamMin=[]  KbParamMax=[]  KtParamMin=[]  KtParamMax=[]  KbOutMin=[]  KbOutMax=[]  KtOutMin=[]  KtOutMax=[]  IntegratorOutMin=[]  IntegratorOutMax=[]  FilterOutMin=[]  FilterOutMax=[]  SumI1OutMin=[]  SumI1OutMax=[]  SumI2OutMin=[]  SumI2OutMax=[]  SumI3OutMin=[]  SumI3OutMax=[]  SumI4OutMin=[]  SumI4OutMax=[]  SumDOutMin=[]  SumDOutMax=[]  DifferentiatorOutMin=[]  DifferentiatorOutMax=[]  FilterDiffOutCoefMin=[]  FilterDiffOutCoefMax=[]  ReciprocalOutMin=[]  ReciprocalOutMax=[]  SumDenOutMin=[]  SumDenOutMax=[]  SumNumOutMin=[]  SumNumOutMax=[]  DivideOutMin=[]  DivideOutMax=[]  UdiffTsProdOutMin=[]  UdiffTsProdOutMax=[]  NTsProdOutMin=[]  NTsProdOutMax=[]  UintegralTsProdOutMin=[]  UintegralTsProdOutMax=[]  UngainTsProdOutMin=[]  UngainTsProdOutMax=[]  ClampingZeroOutDataTypeStr=Inherit: Inherit via back propagation  ClampingZeroOutMin=[]  ClampingZeroOutMax=[]  FilterDenConstantOutDataTypeStr=Inherit: Inherit via back propagation  FilterDenConstantOutMin=[]  FilterDenConstantOutMax=[]  PCopyOutDataTypeStr=Inherit: Inherit via back propagation  PCopyOutMin=[]  PCopyOutMax=[]  NCopyOutDataTypeStr=Inherit: Inherit via back propagation  NCopyOutMin=[]  NCopyOutMax=[]  IntegratorContinuousStateAttributes=''  IntegratorStateMustResolveToSignalObject=off  IntegratorRTWStateStorageClass=Auto  FilterContinuousStateAttributes=''  FilterStateMustResolveToSignalObject=off  FilterRTWStateStorageClass=Auto  ParallelPVariant=InternalParameters  IdealPVariant=Disabled  IVariant=InternalParameters  DVariant=InternalParameters  IntegratorVariant=Continuous  SatVariant=Disabled  AWVariant=Passthrough  PCopyVariant=Disabled  TRVariant=Disabled  FdbkBlocksVariant=Forward  IdealPFdbkVariant=Disabled  SatFdbkVariant=Disabled  DerivativeFilterVariant=ContFilter  NVariant=InternalParameters  NCopyVariant=Disabled  FilterICVariant=InternalICsFilter  IntegratorICVariant=InternalICs  ExternalResetVariant=Disabled  TRSumVariant=Passthrough  SumFdbkVariant=Disabled  SumVariant=Sum_PID  TsampFilterVariant=InternalTs  TsampNgainVariant=Passthrough  TsampIntegralVariant=Disabled_SignalSpec  ExternalSaturationOutDataTypeStr=Inherit: Same as second input
  Pulse Generator : DiscretePulseGenerator  PulseType=Time based  Amplitude=5  Period=40  PulseWidth=50
  Scope{1..7} (7 alike) : Scope
  Step : Step  Time=20  After=5  SampleTime=0
  Sum{1..6} (6 alike) : Sum  Inputs=|+-
  Terminator{2..3,5..8} (6 alike) : Terminator
  Out1 : Outport
  wires:
  PID Controller5/1 -> Mux/1
  Sum5/1 -> PID Controller5/1
  Step/1 -> [xyon]
  [xyon] -> Sum5/1
  PID Controller6/1 -> Mux/2
  Sum6/1 -> PID Controller6/1
  Constant4/1 -> Sum6/1
  [Y] -> Sum6/2
  PID Controller4/1 -> Mux/4
  Sum4/1 -> PID Controller4/1
  Constant3/1 -> Sum4/1
  [beta] -> Sum4/2
  Demux/6 -> Scope6/1, [psi]
  PID Controller3/1 -> Mux/6
  Constant1/1 -> Sum3/1
  Sum3/1 -> PID Controller3/1
  [psi] -> Sum3/2
  [Z] -> Sum1/2
  [X] -> Sum5/2
  PID Controller2/1 -> Mux/5
  [teta] -> Sum2/2
  Constant2/1 -> Sum2/1
  Sum2/1 -> PID Controller2/1
  PID Controller1/1 -> Mux/3
  Demux/3 -> Scope1/1, [Z]
  Demux1/6 -> Terminator3/1
  Demux1/5 -> Terminator2/1
  Sum1/1 -> PID Controller1/1
  Demux1/4 -> Terminator8/1
  Demux1/3 -> Terminator7/1
  Demux1/2 -> Terminator6/1
  Demux1/1 -> Terminator5/1
  Demux/4 -> Scope4/1, [beta]
  Demux/5 -> [teta], Scope5/1
  Demux/2 -> Scope3/1, [Y]
  Demux/1 -> Scope2/1, [X]
  Input/1 -> Demux/1
  Mux/1 -> Demux1/1, Out1/1
  Constant/1 -> Sum1/1
  Pulse Generator/1 -> Scope7/1

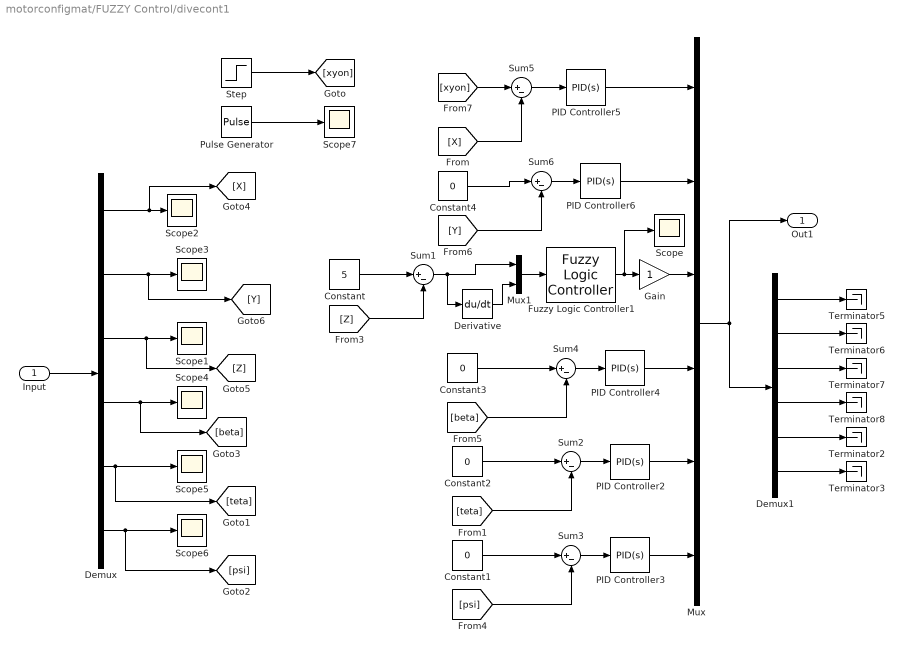
== system motorconfigmat/FUZZY Control/divecont1 ==
  Input : Inport
  Constant : Constant  Value=5
  Constant{1..4} (4 alike) : Constant  Value=0
  Demux : Demux  Outputs=6
  Demux1 : Demux  Outputs=6
  Derivative : Derivative
  Fuzzy Logic Controller1 : fuzblock/Fuzzy Logic  Controller  FIS='FLCbilalebuldu.fis'  OutputSampleNumber=101  DataType=double  FuzzifiedInputs=off  RuleFiringStrengths=off  RuleOutputs=off  AggregatedOutputs=off  SimulateUsing=Interpreted execution  OutOfRangeInputValueMessage=warning  NoRuleFiredMessage=warning  EmptyOutputFuzzySetMessage=warning
  Gain : Gain
  Mux : Mux  Inputs=6
  Mux1 : Mux  Inputs=2
  PID Controller{2..4,6} (4 alike) : slpidlib/PID Controller  Controller=PID  Form=Parallel  TimeDomain=Continuous-time  UseExternalTs=off  SampleTime=-1  IntegratorMethod=Forward Euler  FilterMethod=Forward Euler  ControllerParametersSource=internal  P=0.2  I=0  UseKiTs=off  D=0  N=100  UseFilter=on  TunerSelectOption=Transfer Function Based (PID Tuner App)  InitialConditionSource=internal  InitialConditionForIntegrator=0  InitialConditionForFilter=0  DifferentiatorICPrevScaledInput=0  ExternalReset=none  TrackingMode=off  Kt=1  LimitOutput=off  SatLimitsSource=internal  UpperSaturationLimit=inf  LowerSaturationLimit=-inf  LinearizeAsGain=on  AntiWindupMode=none  Kb=1  LimitIntegrator=off  UpperIntegratorSaturationLimit=inf  LowerIntegratorSaturationLimit=-inf  POutMin=[]  POutMax=[]  IOutMin=[]  IOutMax=[]  DOutMin=[]  DOutMax=[]  NOutMin=[]  NOutMax=[]  SumOutMin=[]  SumOutMax=[]  SaturationOutMin=[]  SaturationOutMax=[]  PParamMin=[]  PParamMax=[]  IParamMin=[]  IParamMax=[]  DParamMin=[]  DParamMax=[]  NParamMin=[]  NParamMax=[]  KbParamMin=[]  KbParamMax=[]  KtParamMin=[]  KtParamMax=[]  KbOutMin=[]  KbOutMax=[]  KtOutMin=[]  KtOutMax=[]  IntegratorOutMin=[]  IntegratorOutMax=[]  FilterOutMin=[]  FilterOutMax=[]  SumI1OutMin=[]  SumI1OutMax=[]  SumI2OutMin=[]  SumI2OutMax=[]  SumI3OutMin=[]  SumI3OutMax=[]  SumI4OutMin=[]  SumI4OutMax=[]  SumDOutMin=[]  SumDOutMax=[]  DifferentiatorOutMin=[]  DifferentiatorOutMax=[]  FilterDiffOutCoefMin=[]  FilterDiffOutCoefMax=[]  ReciprocalOutMin=[]  ReciprocalOutMax=[]  SumDenOutMin=[]  SumDenOutMax=[]  SumNumOutMin=[]  SumNumOutMax=[]  DivideOutMin=[]  DivideOutMax=[]  UdiffTsProdOutMin=[]  UdiffTsProdOutMax=[]  NTsProdOutMin=[]  NTsProdOutMax=[]  UintegralTsProdOutMin=[]  UintegralTsProdOutMax=[]  UngainTsProdOutMin=[]  UngainTsProdOutMax=[]  ClampingZeroOutDataTypeStr=Inherit: Inherit via back propagation  ClampingZeroOutMin=[]  ClampingZeroOutMax=[]  FilterDenConstantOutDataTypeStr=Inherit: Inherit via back propagation  FilterDenConstantOutMin=[]  FilterDenConstantOutMax=[]  PCopyOutDataTypeStr=Inherit: Inherit via back propagation  PCopyOutMin=[]  PCopyOutMax=[]  NCopyOutDataTypeStr=Inherit: Inherit via back propagation  NCopyOutMin=[]  NCopyOutMax=[]  IntegratorContinuousStateAttributes=''  IntegratorStateMustResolveToSignalObject=off  IntegratorRTWStateStorageClass=Auto  FilterContinuousStateAttributes=''  FilterStateMustResolveToSignalObject=off  FilterRTWStateStorageClass=Auto  ParallelPVariant=InternalParameters  IdealPVariant=Disabled  IVariant=InternalParameters  DVariant=InternalParameters  IntegratorVariant=Continuous  SatVariant=Disabled  AWVariant=Passthrough  PCopyVariant=Disabled  TRVariant=Disabled  FdbkBlocksVariant=Forward  IdealPFdbkVariant=Disabled  SatFdbkVariant=Disabled  DerivativeFilterVariant=ContFilter  NVariant=InternalParameters  NCopyVariant=Disabled  FilterICVariant=InternalICsFilter  IntegratorICVariant=InternalICs  ExternalResetVariant=Disabled  TRSumVariant=Passthrough  SumFdbkVariant=Disabled  SumVariant=Sum_PID  TsampFilterVariant=InternalTs  TsampNgainVariant=Passthrough  TsampIntegralVariant=Disabled_SignalSpec  ExternalSaturationOutDataTypeStr=Inherit: Same as second input
  PID Controller5 : slpidlib/PID Controller  Controller=PID  Form=Parallel  TimeDomain=Continuous-time  UseExternalTs=off  SampleTime=-1  IntegratorMethod=Forward Euler  FilterMethod=Forward Euler  ControllerParametersSource=internal  P=0.9  I=0  UseKiTs=off  D=0  N=100  UseFilter=on  TunerSelectOption=Transfer Function Based (PID Tuner App)  InitialConditionSource=internal  InitialConditionForIntegrator=0  InitialConditionForFilter=0  DifferentiatorICPrevScaledInput=0  ExternalReset=none  TrackingMode=off  Kt=1  LimitOutput=off  SatLimitsSource=internal  UpperSaturationLimit=inf  LowerSaturationLimit=-inf  LinearizeAsGain=on  AntiWindupMode=none  Kb=1  LimitIntegrator=off  UpperIntegratorSaturationLimit=inf  LowerIntegratorSaturationLimit=-inf  POutMin=[]  POutMax=[]  IOutMin=[]  IOutMax=[]  DOutMin=[]  DOutMax=[]  NOutMin=[]  NOutMax=[]  SumOutMin=[]  SumOutMax=[]  SaturationOutMin=[]  SaturationOutMax=[]  PParamMin=[]  PParamMax=[]  IParamMin=[]  IParamMax=[]  DParamMin=[]  DParamMax=[]  NParamMin=[]  NParamMax=[]  KbParamMin=[]  KbParamMax=[]  KtParamMin=[]  KtParamMax=[]  KbOutMin=[]  KbOutMax=[]  KtOutMin=[]  KtOutMax=[]  IntegratorOutMin=[]  IntegratorOutMax=[]  FilterOutMin=[]  FilterOutMax=[]  SumI1OutMin=[]  SumI1OutMax=[]  SumI2OutMin=[]  SumI2OutMax=[]  SumI3OutMin=[]  SumI3OutMax=[]  SumI4OutMin=[]  SumI4OutMax=[]  SumDOutMin=[]  SumDOutMax=[]  DifferentiatorOutMin=[]  DifferentiatorOutMax=[]  FilterDiffOutCoefMin=[]  FilterDiffOutCoefMax=[]  ReciprocalOutMin=[]  ReciprocalOutMax=[]  SumDenOutMin=[]  SumDenOutMax=[]  SumNumOutMin=[]  SumNumOutMax=[]  DivideOutMin=[]  DivideOutMax=[]  UdiffTsProdOutMin=[]  UdiffTsProdOutMax=[]  NTsProdOutMin=[]  NTsProdOutMax=[]  UintegralTsProdOutMin=[]  UintegralTsProdOutMax=[]  UngainTsProdOutMin=[]  UngainTsProdOutMax=[]  ClampingZeroOutDataTypeStr=Inherit: Inherit via back propagation  ClampingZeroOutMin=[]  ClampingZeroOutMax=[]  FilterDenConstantOutDataTypeStr=Inherit: Inherit via back propagation  FilterDenConstantOutMin=[]  FilterDenConstantOutMax=[]  PCopyOutDataTypeStr=Inherit: Inherit via back propagation  PCopyOutMin=[]  PCopyOutMax=[]  NCopyOutDataTypeStr=Inherit: Inherit via back propagation  NCopyOutMin=[]  NCopyOutMax=[]  IntegratorContinuousStateAttributes=''  IntegratorStateMustResolveToSignalObject=off  IntegratorRTWStateStorageClass=Auto  FilterContinuousStateAttributes=''  FilterStateMustResolveToSignalObject=off  FilterRTWStateStorageClass=Auto  ParallelPVariant=InternalParameters  IdealPVariant=Disabled  IVariant=InternalParameters  DVariant=InternalParameters  IntegratorVariant=Continuous  SatVariant=Disabled  AWVariant=Passthrough  PCopyVariant=Disabled  TRVariant=Disabled  FdbkBlocksVariant=Forward  IdealPFdbkVariant=Disabled  SatFdbkVariant=Disabled  DerivativeFilterVariant=ContFilter  NVariant=InternalParameters  NCopyVariant=Disabled  FilterICVariant=InternalICsFilter  IntegratorICVariant=InternalICs  ExternalResetVariant=Disabled  TRSumVariant=Passthrough  SumFdbkVariant=Disabled  SumVariant=Sum_PID  TsampFilterVariant=InternalTs  TsampNgainVariant=Passthrough  TsampIntegralVariant=Disabled_SignalSpec  ExternalSaturationOutDataTypeStr=Inherit: Same as second input
  Pulse Generator : DiscretePulseGenerator  PulseType=Time based  Amplitude=5  Period=40  PulseWidth=50
  Scope{,1..7} (8 alike) : Scope
  Step : Step  Time=20  After=5  SampleTime=0
  Sum{1..6} (6 alike) : Sum  Inputs=|+-
  Terminator{2..3,5..8} (6 alike) : Terminator
  Out1 : Outport
  wires:
  Pulse Generator/1 -> Scope7/1
  Constant/1 -> Sum1/1
  Mux/1 -> Out1/1, Demux1/1
  Input/1 -> Demux/1
  Demux/1 -> [X], Scope2/1
  Demux/2 -> [Y], Scope3/1
  Demux/5 -> Scope5/1, [teta]
  Demux/4 -> [beta], Scope4/1
  Demux1/1 -> Terminator5/1
  Demux1/2 -> Terminator6/1
  Demux1/3 -> Terminator7/1
  Demux1/4 -> Terminator8/1
  Demux1/5 -> Terminator2/1
  Demux1/6 -> Terminator3/1
  Demux/3 -> [Z], Scope1/1
  Sum2/1 -> PID Controller2/1
  Constant2/1 -> Sum2/1
  [teta] -> Sum2/2
  PID Controller2/1 -> Mux/5
  [X] -> Sum5/2
  [Z] -> Sum1/2
  [psi] -> Sum3/2
  Sum3/1 -> PID Controller3/1
  Constant1/1 -> Sum3/1
  PID Controller3/1 -> Mux/6
  Demux/6 -> [psi], Scope6/1
  [beta] -> Sum4/2
  Constant3/1 -> Sum4/1
  Sum4/1 -> PID Controller4/1
  PID Controller4/1 -> Mux/4
  [Y] -> Sum6/2
  Constant4/1 -> Sum6/1
  Sum6/1 -> PID Controller6/1
  PID Controller6/1 -> Mux/2
  [xyon] -> Sum5/1
  Step/1 -> [xyon]
  Sum5/1 -> PID Controller5/1
  PID Controller5/1 -> Mux/1
  Sum1/1 -> Derivative/1, Mux1/1
  Derivative/1 -> Mux1/2
  Mux1/1 -> Fuzzy Logic Controller1/1
  Fuzzy Logic Controller1/1 -> Scope/1, Gain/1
  Gain/1 -> Mux/3

== system motorconfigmat/Subsystem/CA ==
  velociyC : Inport
  velocity : Inport  Port=2
  Add : Sum  Inputs=+-
  MATLAB Function : MATLAB Function  TreatAsAtomicUnit=on
  CA : Outport
  wires:
  MATLAB Function/1(y) -> CA/1
  velociyC/1 -> Add/2
  velocity/1 -> Add/1
  Add/1 -> MATLAB Function/1(Vw)

== system motorconfigmat/Subsystem/CRB ==
  velo : Inport
  MATLAB Function : MATLAB Function  TreatAsAtomicUnit=on
  y : Outport
  wires:
  velo/1 -> MATLAB Function/1(V)
  MATLAB Function/1(y) -> y/1

== system motorconfigmat/Subsystem/Damp ==
  veloC : Inport
  velu : Inport  Port=2
  Add : Sum  Inputs=+-
  MATLAB Function : MATLAB Function  TreatAsAtomicUnit=on
  y : Outport
  wires:
  MATLAB Function/1(y) -> y/1
  velu/1 -> Add/1
  veloC/1 -> Add/2
  Add/1 -> MATLAB Function/1(Vw)

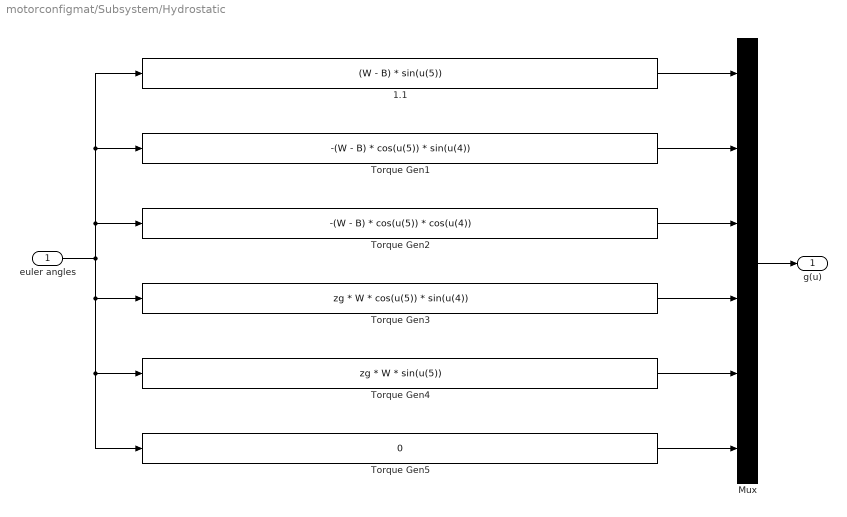
== system motorconfigmat/Subsystem/Hydrostatic ==
  euler angles : Inport
  1.1 : Fcn  Expr=(W - B) * sin(u(5))
  Mux : Mux  Inputs=6
  Torque Gen1 : Fcn  Expr=-(W - B) * cos(u(5)) * sin(u(4))
  Torque Gen2 : Fcn  Expr=-(W - B) * cos(u(5)) * cos(u(4))
  Torque Gen3 : Fcn  Expr=zg * W * cos(u(5)) * sin(u(4))
  Torque Gen4 : Fcn  Expr=zg * W * sin(u(5))
  Torque Gen5 : Fcn  Expr=0
  g(u) : Outport
  wires:
  euler angles/1 -> 1.1/1, Torque Gen1/1, Torque Gen2/1, Torque Gen5/1, Torque Gen4/1, Torque Gen3/1
  Torque Gen3/1 -> Mux/4
  Torque Gen2/1 -> Mux/3
  Torque Gen1/1 -> Mux/2
  1.1/1 -> Mux/1
  Torque Gen4/1 -> Mux/5
  Torque Gen5/1 -> Mux/6
  Mux/1 -> g(u)/1

== system motorconfigmat/Subsystem/MA ==
  veloC : Inport
  MATLAB Function : MATLAB Function  TreatAsAtomicUnit=on
  y : Outport
  wires:
  MATLAB Function/1(y) -> y/1
  veloC/1 -> MATLAB Function/1(accelW)

== system motorconfigmat/Subsystem/inv MA and MRB ==
  u : Inport
  MA ve MRB : MATLAB Function  TreatAsAtomicUnit=on
  MRB sadece : MATLAB Function  Commented=on  TreatAsAtomicUnit=on
  accel : Outport
  wires:
  u/1 -> MA ve MRB/1(u)
  MA ve MRB/1(y) -> accel/1

== matlab function motorconfigmat/Subsystem/CA/MATLAB Function ==
  data: Vw input; y output
function y = fcn(Vw)

u = Vw(1);
v = Vw(2);
w = Vw(3);

p = Vw(4);
q = Vw(5);
r = Vw(6);

Xu_dot = -5.5;   % Surge direction
Yv_dot = -12.7;  % Sway direction
Zw_dot = -14.57; % Heave direction

Kp_dot = -0.12;  % Roll moment
Mq_dot = -0.12;  % Pitch moment
Nr_dot = -0.12;  % Yaw moment



% ek kütle corriolis Matrisin tanımlanması
    CA = [
        0,        0,          0,        0,          Zw_dot*w,  0        ;
        0,        0,          0,       -Zw_dot*w,   0,         -Xu_dot*u;
        0,        0,          0,       -Yv_dot*v,   Xu_dot*u,  0        ;
        0,       -Zw_dot*w,  Yv_dot*v,  0,         -Nr_dot*r,  Mq_dot*q ;
        Zw_dot*w, 0,        -Xu_dot*u,  Nr_dot*r,   0,        -Kp_dot*p ;
       -Yv_dot*v, Xu_dot*u,   0,       -Mq_dot*q,   Kp_dot*p,  0        ;
    ];


y = CA * Vw ;

== matlab function motorconfigmat/Control allocation/MATLAB Function ==
  data: T input; tau input; u output
function u = fcn(T, tau)
K = [40 40 40 40 40 40 40 40];
thurustcof = diag(K);
Tplus= T' * inv(T*T');

u = inv(thurustcof) * Tplus * tau;

== matlab function motorconfigmat/Control allocation/MATLAB Function1 ==
  data: F1 input; thrust1 output
function thrust1 = fcn(F1)

% T1
lx1 = 156 / 1000;  % metre
ly1 = 111 / 1000;  % metre
lz1 = 85 / 1000;   % metre
F1q = pi/4;

Fx = F1 * cos(F1q);
Fy = -F1 * sin(F1q);
Fz = 0;

% Matrisin tanımlanması
forces_and_moments = [
    Fx;                  % Kuvvet: x bileşeni
    Fy;                  % Kuvvet: y bileşeni
    Fz;                  % Kuvvet: z bileşeni
    Fz*ly1 - Fy*lz1;    % Moment: x ekseni etrafında
    Fx*lz1 - Fz*lx1;    % Moment: y ekseni etrafında
    Fy*lx1 - Fx*ly1     % Moment: z ekseni etrafında
];
% Sonuçların görüntülenmesi
%disp('Forces and Moments Matrix:');
%disp(forces_and_moments);

thrust1 = forces_and_moments;

== matlab function motorconfigmat/Control allocation/MATLAB Function2 ==
  data: F2 input; thrust2 output
function thrust2 = fcn(F2)

% T2
lx2 = 156 / 1000;  % metre
ly2 = -111 / 1000; % metre
lz2 = 85 / 1000;   % metre
F2q = pi/4;

Fx = F2 * cos(F2q);
Fy = F2 * sin(F2q);
Fz = 0;

% Matrisin tanımlanması
forces_and_moments = [
    Fx;                  % Kuvvet: x bileşeni
    Fy;                  % Kuvvet: y bileşeni
    Fz;                  % Kuvvet: z bileşeni
    Fz*ly2 - Fy*lz2;    % Moment: x ekseni etrafında
    Fx*lz2 - Fz*lx2;    % Moment: y ekseni etrafında
    (Fy*lx2 - Fx*ly2)     % Moment: z ekseni etrafında burda liva farklı yapmıs
];
% Sonuçların görüntülenmesi
%disp('Forces and Moments Matrix:');
%disp(forces_and_moments);

thrust2 = forces_and_moments;

== matlab function motorconfigmat/Control allocation/MATLAB Function3 ==
  data: F3 input; thrust3 output
function thrust3 = fcn(F3)

% T3
lx3 = -156 / 1000; % metre
ly3 = 111 / 1000;  % metre
lz3 = 85 / 1000;   % metre
F3q = pi/4;


Fx = -F3 * cos(F3q);
Fy = -F3 * sin(F3q);
Fz = 0;

% Matrisin tanımlanması
forces_and_moments = [
    Fx;                  % Kuvvet: x bileşeni
    Fy;                  % Kuvvet: y bileşeni
    Fz;                  % Kuvvet: z bileşeni
    Fz*ly3 - Fy*lz3;    % Moment: x ekseni etrafında
    Fx*lz3 - Fz*lx3;    % Moment: y ekseni etrafında
    (Fy*lx3 - Fx*ly3)     % Moment: z ekseni etrafında burda da bi fark var
];
% Sonuçların görüntülenmesi
%disp('Forces and Moments Matrix:');
%disp(forces_and_moments);

thrust3 = forces_and_moments;
